simulink model "Environment_PMWS"  (R2018a)
settings: Solver=FixedStepAuto  StartTime=0.0  StopTime=660  FixedStep=0.001  EnableMultiTasking=on
PreLoadFcn:
  | Environment_PreLoad
model workspace (MAT data in the model file):
  JC08_speed = [0 0 0 0 0 0 0 0 0 0 0 0 ... (1205 elements, 1205x1)]
  JC08_time = [0 1 2 3 4 5 6 7 8 9 10 11 ... (1205 elements, 1205x1)]
undefined symbols (not defined in the file or in its folder): sigbuilder_block
Description:
  | Ver1 ：
  | ブレーキモデル組み込み前に、Tireブロックから車輪速を出力できるように
  | Simscapeブロック変更したものを組み込み動作確認
  | 
  | Ver2　：
  | ブレーキモデルを組み込み。シミュレーション時間大のためソルバを
  | ode15s -> ode23tに変更して動作確認。ＯＫ
  | 
  | 
  | Ver3 ：
  | センサ（相当）信号と制御信号を整理、ただし、ブレーキモデルはコントローラ込で
  | ＰＴモデル内のまま
  | 
  | Ver4：
  | ブレーキモデル内のデータログ関連のブロックを削除し、シミュレーション時間を
  | 短縮できたので、ソルバはode15sのままにしておく。
  | DriverSubsytem追加（中身は、Signla Builderのまま）
  | 
  | Ver5：
  | Coolingモデルの追加。信号の接続はSimulink信号。
  | 
  | Ver6：
  | 暫定で、Coolingモデルの水温を読み込んで、エンジンフリクションを変化させる。
  | ただし、フリクションは0に設定し、エンジン出力には影響なし。
  | 代数ループの影響をみるため。Simulink信号に変換したうえで接続
  | －＞動作せず
  | 
  | Ver7：
  | Simscape信号のまま接続。動作問題なし。
  | 
  | Ver10：
  | Driverモデルの組み込み、10-15modeでの走行確認。
  | ブレーキ協調コントローラがないため、ブレーキモデルへのブレーキ指示信号未接続。
  | 減速はモータのみ。
  | 
  | 
  | 
  | （今後の予定）
  | エンジンクーリングモデルの追加、エンジンモデル入れ替え
  | HEVシステムの組み替え
  | Inverterモデルの接続検討
settings Model: Creator=1442442  LastModifiedBy=E00026
settings SolverCC: MaxOrder=2  ZeroCrossControl=DisableAll
settings DataIOCC: SaveFormat=Array  SignalLoggingSaveFormat=ModelDataLogs  SaveOutput=off  SignalLogging=off  DSMLogging=off  SaveTime=off
settings OptimizationCC: ExpressionDepthLimit=2147483647  LifeSpan=inf
settings DebuggingCC: AlgebraicLoopMsg=error  UnderspecifiedInitializationDetection=Classic  MergeDetectMultiDrivingBlocksExec=none  FcnCallInpInsideContextMsg=warning  StateNameClashWarn=warning  SFUnexpectedBacktrackingDiag=warning  SFNoUnconditionalDefaultTransitionDiag=warning  SFExecutionAtInitializationDiag=none
settings HardwareCC: ProdBitPerPointer=32  ProdBitPerSizeT=32  ProdBitPerPtrDiffT=32  ProdLargestAtomicFloat=None  ProdIntDivRoundTo=Undefined  ProdEndianess=Unspecified  ProdWordSize=32  ProdHWDeviceType=32-bit Generic
settings ModelReferenceCC: PropagateSignalLabelsOutOfModel=off
settings CodeAppCC: StateflowObjectComments=on
settings GRTTargetCC: TargetLangStandard=C89/C90 (ANSI)  GeneratePreprocessorConditionals=Disable all  CombineOutputUpdateFcns=off  GRTInterface=on
settings ConfigComp: CovMetricSettings=dw  CovHtmlReporting=on  CovSaveCumulativeToWorkspaceVar=on  CovSaveSingleToWorkspaceVar=on  CovExternalEMLEnable=off  CovSFcnEnable=off
settings SimscapeCC: SimscapeNormalizeSystem=off  SimscapeLogSimulationStatistics=on  SimscapeLogOpenViewer=on  SimscapeLogLimitData=off

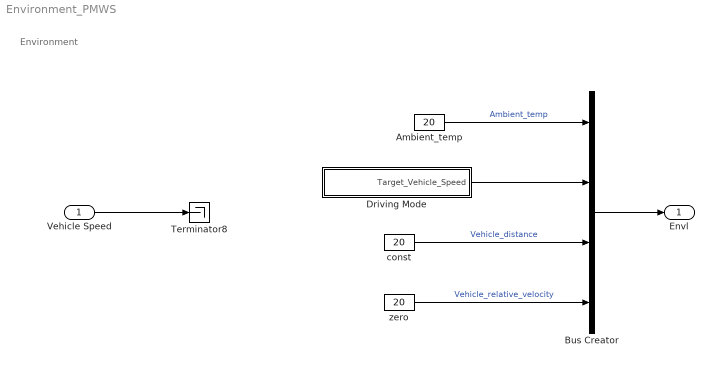
== system Environment_PMWS ==
  note: Environment
  Vehicle Speed : Inport
  Ambient_temp : Constant  Value=20
  Bus Creator : BusCreator  Inputs=4  OutDataTypeStr=Bus: Environment_Bus
      settings: AttributesFormatString=%<OutDataTypeStr>
  Driving Mode : Subsystem
  Terminator8 : Terminator
  const : Constant  Value=20
  zero : Constant  Value=20
  Envl : Outport  OutDataTypeStr=Bus: Environment_Bus
      settings: AttributesFormatString=%<OutDataTypeStr>
  wires:
  Bus Creator/1 -> Envl/1
  Ambient_temp/1 -> Bus Creator/1  "Ambient_temp"
  Driving Mode/1(Target_Vehicle_Speed) -> Bus Creator/2
  Vehicle Speed/1 -> Terminator8/1
  const/1 -> Bus Creator/3  "Vehicle_distance"
  zero/1 -> Bus Creator/4  "Vehicle_relative_velocity"

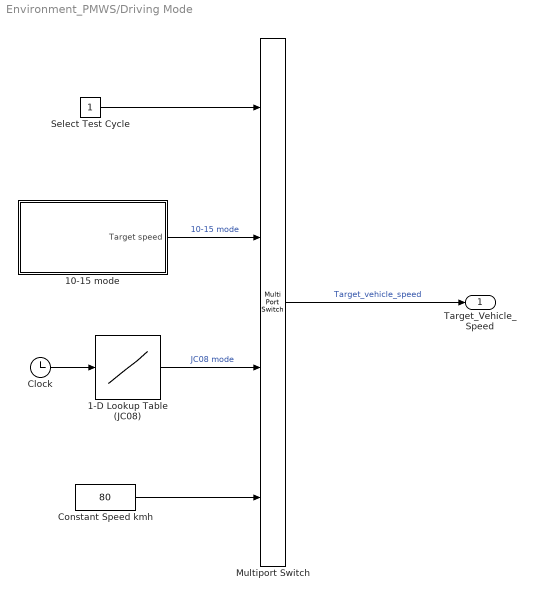
== system Environment_PMWS/Driving Mode ==
  1-D Lookup Table (JC08) : Lookup_n-D  NumberOfTableDimensions=1  BreakpointsForDimension1=JC08_time  Table=JC08_speed  ExtrapMethod=Clip  InternalRulePriority=Speed  RndMeth=Simplest  InputSameDT=on
  "10-15 mode " : Subsystem  Tag=STV Subsys  LoadFcn=sigbuilder_block('load');  StartFcn=sigbuilder_block('start');  StopFcn=sigbuilder_block('stop');  ClipboardFcn=sigbuilder_block('clipboard');  mask(Sigbuilder block){tuvar=[0:10]}
      mask help: Sigbuilder GUI
      mask init:
      | if ~strcmp(get_param(bdroot(gcbh),'SimulationStatus'),'stopped') tuvar = sigbuilder_block('maskInit'); end
      settings: CopyFcn=sigbuilder_block('copy');  DeleteFcn=sigbuilder_block('delete');  ModelCloseFcn=sigbuilder_block('modelClose');  PreSaveFcn=sigbuilder_block('preSave');  PauseFcn=sigbuilder_block('pause')  ContinueFcn=sigbuilder_block('continue')  NameChangeFcn=sigbuilder_block('namechange');  OpenFcn=sigbuilder_block('open',[303 108.75 551.25 359.25 ]);  CloseFcn=sigbuilder_block('close');
      mask Display: plot(0, 0, 100, 100,[2, 2, 32, 32, 2], [68, 8, 8, 68, 68],[32, 2], [38, 38], [32, 19, 2],[53, 60, 44], [32, 17, 17, 2],[16, 16, 31, 31]);txt = getActiveGroup(gcbh);text(2, 100, txt,'verticalAlignment', 'top');
  Clock : Clock
  Constant Speed kmh : Constant  Value=80
  Multiport Switch : MultiPortSwitch
  Select Test Cycle : Constant
  Target_Vehicle_Speed : Outport  Unit=km/h
  wires:
  Multiport Switch/1 -> Target_Vehicle_Speed/1  "Target_vehicle_speed"
  Clock/1 -> 1-D Lookup Table (JC08)/1
  "10-15 mode "/1(Target speed) -> Multiport Switch/2  "10-15 mode"
  Select Test Cycle/1 -> Multiport Switch/1
  1-D Lookup Table (JC08)/1 -> Multiport Switch/3  "JC08 mode"
  Constant Speed kmh/1 -> Multiport Switch/4

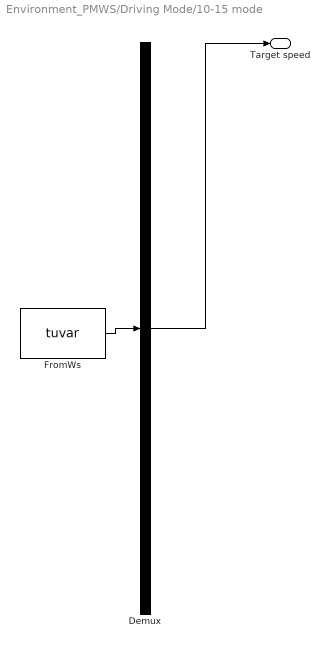
== system Environment_PMWS/Driving Mode/10-15 mode  ==
  Demux : Demux  Tag=STV Demux  Outputs=1
  FromWs : FromWorkspace  Tag=STV FromWs  VariableName=tuvar  SampleTime=0
      SigBuilderData=|
      | common.afterFinalStr = 'Extrapolate'
      | common.sampleTime = '0'
      | dataSet.timeRange = [0 660]
      | dataSet.name = '10-15 Mode Cycle'
      | sbobj.Groups.Name = '10-15 Mode Cycle'
      | sbobj.Groups.Signals.Name = 'Target speed'
      | sbobj.Groups.Signals.XData = [0 44 51 66 73 89 103 118 128 130 142 152 159 179 186 201 208 224 238 253 263 265 277 287 294 314 321 336 343 359 373 388 398 400 412 422 429 494 512 524 528 532 548 558 569 579 589 593 615 620 640 650 660]
      | sbobj.Groups.Signals.YData = [0 0 20 20 0 0 40 40 20 20 40 20 0 0 20 20 0 0 40 40 20 20 40 20 0 0 20 20 0 0 40 40 20 20 40 20 0 0 50 50 40 40 60 60 70 70 50 50 70 70 30 0 0]
      | sbobj.Groups.TimeRange = [0 660]
  Target speed : Outport  Tag=STV Outport
  wires:
  FromWs/1 -> Demux/1
  Demux/1 -> Target speed/1
